simulink library "xpcueilib"  (Simulink 6.0)
settings: Solver=ode45  SolverMode=SingleTasking  StartTime=0.0  StopTime=10.0  RelTol=1e-3
(part 2 of 2)

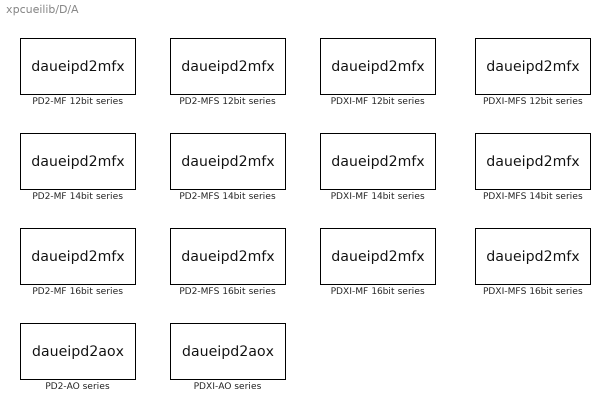
== system xpcueilib/D/A ==
  PD2-AO series : S-Function  InitFcn=muei  FunctionName=daueipd2aox  Parameters=channel, reset, initValue, sampletime, pcislot, boardType, board, devName  mask(ueipd2ao16_da_6){boardtypein=PD2-AO-8/16, channel=[1], reset=[1], initValue=[0], sampletime=0.001, pcislot=-1}
      mask prompts: boardtypein "Board type:"; channel "Channel vector:"; reset "Reset vector:"; initValue "Initial value vector:"; pcislot "PCI slot (-1: autosearch):"
      mask help:
      | PD2-AO series
      | United Electronic Industries
      | Analog Output
      mask init:
      | [board, boardType, devName, reset, initValue, maskdisplay, maskdescription]= mdaueipd2aox(boardtypein, channel, reset, initValue, pcislot);
      | set_param(gcb,'MaskDescription',maskdescription);
      | set_param(gcb,'MaskDisplay',maskdisplay);
      mask Help: helpview(fullfile(docroot, 'mapfiles', 'xpc.map'), 'UEI_PD2-AO-series_DA')
      mask StyleString: popup(PD2-AO-8/16|PD2-AO-16/16|PD2-AO-32/16|PD2-AO-96/16),edit,edit,edit,edit,edit
      mask Display: disp('PD2-AO-8/16\nUEI\nAnalog Output');port_label('input',1,'1');
  PD2-MF 12bit series : S-Function  InitFcn=muei  FunctionName=daueipd2mfx  Parameters=channel, reset, initValue, sampletime, pcislot, boardType, board, devName  mask(ueipd2mf12_da_6){boardtypein=PD2-MF-16-1M/12L, channel=[1], reset=[1], initValue=[0], sampletime=0.001, pcislot=-1}
      mask prompts: boardtypein "Board type:"; channel "Channel vector:"; reset "Reset vector:"; initValue "Initial value vector:"; pcislot "PCI slot (-1: autosearch):"
      mask help:
      | PD2-MF 12bit series
      | United Electronic Industries
      | Analog Output
      mask init: same as xpcueilib/D/A/PD2-AO series
      mask Help: helpview(fullfile(docroot, 'mapfiles', 'xpc.map'), 'UEI_PD2-MF-12bit-series_DA')
      mask StyleString: popup(PD2-MF-16-1M/12L|PD2-MF-16-1M/12H|PD2-MF-64-1M/12L|PD2-MF-64-1M/12H),edit,edit,edit,edit,edit
      mask Display: disp('PD2-MF-16-1M/12L\nUEI\nAnalog Output');port_label('input',1,'1');
  PD2-MF 14bit series : S-Function  InitFcn=muei  FunctionName=daueipd2mfx  Parameters=channel, reset, initValue, sampletime, pcislot, boardType, board, devName  mask(ueipd2mf14_da_6){boardtypein=PD2-MF-16-400/14L, channel=[1], reset=[1], initValue=[0], sampletime=0.001, pcislot=-1}
      mask prompts: boardtypein "Board type:"; channel "Channel vector:"; reset "Reset vector:"; initValue "Initial value vector:"; pcislot "PCI slot (-1: autosearch):"
      mask help:
      | PD2-MF 14bit series
      | United Electronic Industries
      | Analog Output
      mask init: same as xpcueilib/D/A/PD2-AO series
      mask Help: helpview(fullfile(docroot, 'mapfiles', 'xpc.map'), 'UEI_PD2-MF-14bit-series_DA')
      mask StyleString: popup(PD2-MF-16-400/14L|PD2-MF-16-400/14H|PD2-MF-64-400/14L|PD2-MF-64-400/14H|PD2-MF-16-800/14L|PD2-MF-16-800/14H|PD2-MF-64-800/14L|PD2-MF-64-800/14H|PD2-MF-16-2M/14L|PD2-MF-16-2M/14H|PD2-MF-64-2M/14L|PD2-MF-64-2M/14H),edit,edit,edit,edit,edit
      mask Display: disp('PD2-MF-16-400/14L\nUEI\nAnalog Output');port_label('input',1,'1');
  PD2-MF 16bit series : S-Function  InitFcn=muei  FunctionName=daueipd2mfx  Parameters=channel, reset, initValue, sampletime, pcislot, boardType, board, devName  mask(ueipd2mf16_da_6){boardtypein=PD2-MF-16-333/16H, channel=[1], reset=[1], initValue=[0], sampletime=0.001, pcislot=-1}
      mask prompts: boardtypein "Board type:"; channel "Channel vector:"; reset "Reset vector:"; initValue "Initial value vector:"; pcislot "PCI slot (-1: autosearch):"
      mask help:
      | PD2-MF 16bit series
      | United Electronic Industries
      | Analog Output
      mask init: same as xpcueilib/D/A/PD2-AO series
      mask Help: helpview(fullfile(docroot, 'mapfiles', 'xpc.map'), 'UEI_PD2-MF-16bit-series_DA')
      mask StyleString: popup(PD2-MF-16-50/16L|PD2-MF-16-50/16H|PD2-MF-64-50/16L|PD2-MF-64-50/16H|PD2-MF-16-150/16L|PD2-MF-16-150/16H|PD2-MF-64-150/16L|PD2-MF-64-150/16H|PD2-MF-16-333/16L|PD2-MF-16-333/16H|PD2-MF-64-333/16L|PD2-MF-64-333/16H|PD2-MF-16-500/16L|PD2-MF-16-500/16H|PD2-MF-64-500/16L|PD2-MF-64-500/16H),edit,edit,edit,edit,edit
      mask Display: disp('PD2-MF-16-333/16H\nUEI\nAnalog Output');port_label('input',1,'1');
  PD2-MFS 12bit series : S-Function  InitFcn=muei  FunctionName=daueipd2mfx  Parameters=channel, reset, initValue, sampletime, pcislot, boardType, board, devName  mask(ueipd2mfs12_da_6){boardtypein=PD2-MFS-4-1M/12, channel=[1], reset=[1], initValue=[0], sampletime=0.001, pcislot=-1}
      mask prompts: boardtypein "Board type:"; channel "Channel vector:"; reset "Reset vector:"; initValue "Initial value vector:"; pcislot "PCI slot (-1: autosearch):"
      mask help:
      | PD2-MFS 12bit series
      | United Electronic Industries
      | Analog Output
      mask init: same as xpcueilib/D/A/PD2-AO series
      mask Help: helpview(fullfile(docroot, 'mapfiles', 'xpc.map'), 'UEI_PD2-MFS-12bit-series_DA')
      mask StyleString: popup(PD2-MFS-4-1M/12|PD2-MFS-4-1M/12DG|PD2-MFS-4-1M/12H|PD2-MFS-8-1M/12|PD2-MFS-8-1M/12DG|PD2-MFS-8-1M/12H),edit,edit,edit,edit,edit
      mask Display: disp('PD2-MFS-4-1M/12\nUEI\nAnalog Output');port_label('input',1,'1');
  PD2-MFS 14bit series : S-Function  InitFcn=muei  FunctionName=daueipd2mfx  Parameters=channel, reset, initValue, sampletime, pcislot, boardType, board, devName  mask(ueipd2mfs14_da_6){boardtypein=PD2-MFS-4-500/14, channel=[1], reset=[1], initValue=[0], sampletime=0.001, pcislot=-1}
      mask prompts: boardtypein "Board type:"; channel "Channel vector:"; reset "Reset vector:"; initValue "Initial value vector:"; pcislot "PCI slot (-1: autosearch):"
      mask help:
      | PD2-MFS 14bit series
      | United Electronic Industries
      | Analog Output
      mask init: same as xpcueilib/D/A/PD2-AO series
      mask Help: helpview(fullfile(docroot, 'mapfiles', 'xpc.map'), 'UEI_PD2-MFS-14bit-series_DA')
      mask StyleString: popup(PD2-MFS-4-500/14|PD2-MFS-4-500/14DG|PD2-MFS-4-500/14H|PD2-MFS-8-500/14|PD2-MFS-8-500/14DG|PD2-MFS-8-500/14H|PD2-MFS-4-800/14|PD2-MFS-4-800/14DG|PD2-MFS-4-800/14H|PD2-MFS-8-800/14|PD2-MFS-8-800/14DG|PD2-MFS-8-800/14H|PD2-MFS-4-2M/14|PD2-MFS-4-2M/14DG|PD2-MFS-4-2M/14H|PD2-MFS-8-2M/14|PD2-MFS-8-2M/14DG|PD2-MFS-8-2M/14H),edit,edit,edit,edit,edit
      mask Display: disp('PD2-MFS-4-500/14\nUEI\nAnalog Output');port_label('input',1,'1');
  PD2-MFS 16bit series : S-Function  InitFcn=muei  FunctionName=daueipd2mfx  Parameters=channel, reset, initValue, sampletime, pcislot, boardType, board, devName  mask(ueipd2mfs16_da_6){boardtypein=PD2-MFS-4-300/16, channel=[1], reset=[1], initValue=[0], sampletime=0.001, pcislot=-1}
      mask prompts: boardtypein "Board type:"; channel "Channel vector:"; reset "Reset vector:"; initValue "Initial value vector:"; pcislot "PCI slot (-1: autosearch):"
      mask help:
      | PD2-MFS 16bit series
      | United Electronic Industries
      | Analog Output
      mask init: same as xpcueilib/D/A/PD2-AO series
      mask Help: helpview(fullfile(docroot, 'mapfiles', 'xpc.map'), 'UEI_PD2-MFS-16bit-series_DA')
      mask StyleString: popup(PD2-MFS-4-300/16|PD2-MFS-4-300/16DG|PD2-MFS-4-300/16H|PD2-MFS-8-300/16|PD2-MFS-8-300/16DG|PD2-MFS-8-300/16H|PD2-MFS-4-500/16|PD2-MFS-4-500/16DG|PD2-MFS-4-500/16H|PD2-MFS-8-500/16|PD2-MFS-8-500/16DG|PD2-MFS-8-500/16H),edit,edit,edit,edit,edit
      mask Display: disp('PD2-MFS-4-300/16\nUEI\nAnalog Output');port_label('input',1,'1');
  PDXI-AO series : S-Function  InitFcn=muei  FunctionName=daueipd2aox  Parameters=channel, reset, initValue, sampletime, pcislot, boardType, board, devName  mask(ueipdxiao16_da_6){boardtypein=PDXI-AO-8/16, channel=[1], reset=[1], initValue=[0], sampletime=0.001, pcislot=-1}
      mask prompts: boardtypein "Board type:"; channel "Channel vector:"; reset "Reset vector:"; initValue "Initial value vector:"; pcislot "PCI slot (-1: autosearch):"
      mask help:
      | PDXI-AO series
      | United Electronic Industries
      | Analog Output
      mask init: same as xpcueilib/D/A/PD2-AO series
      mask Help: helpview(fullfile(docroot, 'mapfiles', 'xpc.map'), 'UEI_PDXI-AO-series_DA')
      mask StyleString: popup(PDXI-AO-8/16|PDXI-AO-16/16|PDXI-AO-32/16|PDXI-AO-96/16),edit,edit,edit,edit,edit
      mask Display: disp('PDXI-AO-8/16\nUEI\nAnalog Output');port_label('input',1,'1');
  PDXI-MF 12bit series : S-Function  InitFcn=muei  FunctionName=daueipd2mfx  Parameters=channel, reset, initValue, sampletime, pcislot, boardType, board, devName  mask(ueipdximf12_da_6){boardtypein=PDXI-MF-16-1M/12L, channel=[1], reset=[1], initValue=[0], sampletime=0.001, pcislot=-1}
      mask prompts: boardtypein "Board type:"; channel "Channel vector:"; reset "Reset vector:"; initValue "Initial value vector:"; pcislot "PCI slot (-1: autosearch):"
      mask help:
      | PDXI-MF 12bit series
      | United Electronic Industries
      | Analog Output
      mask init: same as xpcueilib/D/A/PD2-AO series
      mask Help: helpview(fullfile(docroot, 'mapfiles', 'xpc.map'), 'UEI_PDXI-MF-12bit-series_DA')
      mask StyleString: popup(PDXI-MF-16-1M/12L|PDXI-MF-16-1M/12H|PDXI-MF-64-1M/12L|PDXI-MF-64-1M/12H),edit,edit,edit,edit,edit
      mask Display: disp('PDXI-MF-16-1M/12L\nUEI\nAnalog Output');port_label('input',1,'1');
  PDXI-MF 14bit series : S-Function  InitFcn=muei  FunctionName=daueipd2mfx  Parameters=channel, reset, initValue, sampletime, pcislot, boardType, board, devName  mask(ueipdximf14_da_6){boardtypein=PDXI-MF-16-400/14L, channel=[1], reset=[1], initValue=[0], sampletime=0.001, pcislot=-1}
      mask prompts: boardtypein "Board type:"; channel "Channel vector:"; reset "Reset vector:"; initValue "Initial value vector:"; pcislot "PCI slot (-1: autosearch):"
      mask help:
      | PDXI-MF 14bit series
      | United Electronic Industries
      | Analog Output
      mask init: same as xpcueilib/D/A/PD2-AO series
      mask Help: helpview(fullfile(docroot, 'mapfiles', 'xpc.map'), 'UEI_PDXI-MF-14bit-series_DA')
      mask StyleString: popup(PDXI-MF-16-400/14L|PDXI-MF-16-400/14H|PDXI-MF-64-400/14L|PDXI-MF-64-400/14H|PDXI-MF-16-800/14L|PDXI-MF-16-800/14H|PDXI-MF-64-800/14L|PDXI-MF-64-800/14H|PDXI-MF-16-2M/14L|PDXI-MF-16-2M/14H|PDXI-MF-64-2M/14L|PDXI-MF-64-2M/14H),edit,edit,edit,edit,edit
      mask Display: disp('PDXI-MF-16-400/14L\nUEI\nAnalog Output');port_label('input',1,'1');
  PDXI-MF 16bit series : S-Function  InitFcn=muei  FunctionName=daueipd2mfx  Parameters=channel, reset, initValue, sampletime, pcislot, boardType, board, devName  mask(ueipdximf16_da_6){boardtypein=PDXI-MF-16-333/16H, channel=[1], reset=[1], initValue=[0], sampletime=0.001, pcislot=-1}
      mask prompts: boardtypein "Board type:"; channel "Channel vector:"; reset "Reset vector:"; initValue "Initial value vector:"; pcislot "PCI slot (-1: autosearch):"
      mask help:
      | PDXI-MF 16bit series
      | United Electronic Industries
      | Analog Output
      mask init: same as xpcueilib/D/A/PD2-AO series
      mask Help: helpview(fullfile(docroot, 'mapfiles', 'xpc.map'), 'UEI_PDXI-MF-16bit-series_DA')
      mask StyleString: popup(PDXI-MF-16-50/16L|PDXI-MF-16-50/16H|PDXI-MF-64-50/16L|PDXI-MF-64-50/16H|PDXI-MF-16-150/16L|PDXI-MF-16-150/16H|PDXI-MF-64-150/16L|PDXI-MF-64-150/16H|PDXI-MF-16-333/16L|PDXI-MF-16-333/16H|PDXI-MF-64-333/16L|PDXI-MF-64-333/16H|PDXI-MF-16-500/16L|PDXI-MF-16-500/16H|PDXI-MF-64-500/16L|PDXI-MF-64-500/16H),edit,edit,edit,edit,edit
      mask Display: disp('PDXI-MF-16-333/16H\nUEI\nAnalog Output');port_label('input',1,'1');
  PDXI-MFS 12bit series : S-Function  InitFcn=muei  FunctionName=daueipd2mfx  Parameters=channel, reset, initValue, sampletime, pcislot, boardType, board, devName  mask(ueipd2mfs12_da_6){boardtypein=PDXI-MFS-4-1M/12, channel=[1], reset=[1], initValue=[0], sampletime=0.001, pcislot=-1}
      mask prompts: boardtypein "Board type:"; channel "Channel vector:"; reset "Reset vector:"; initValue "Initial value vector:"; pcislot "PCI slot (-1: autosearch):"
      mask help:
      | PD2-MFS 12bit series
      | United Electronic Industries
      | Analog Output
      mask init: same as xpcueilib/D/A/PD2-AO series
      mask Help: helpview(fullfile(docroot, 'mapfiles', 'xpc.map'), 'UEI_PDXI-MFS-12bit-series_DA')
      mask StyleString: popup(PDXI-MFS-4-1M/12|PDXI-MFS-4-1M/12DG|PDXI-MFS-4-1M/12H|PDXI-MFS-8-1M/12|PDXI-MFS-8-1M/12DG|PDXI-MFS-8-1M/12H),edit,edit,edit,edit,edit
      mask Display: disp('PDXI-MFS-4-1M/12\nUEI\nAnalog Output');port_label('input',1,'1');
  PDXI-MFS 14bit series : S-Function  InitFcn=muei  FunctionName=daueipd2mfx  Parameters=channel, reset, initValue, sampletime, pcislot, boardType, board, devName  mask(ueipd2mfs14_da_6){boardtypein=PDXI-MFS-4-500/14, channel=[1], reset=[1], initValue=[0], sampletime=0.001, pcislot=-1}
      mask prompts: boardtypein "Board type:"; channel "Channel vector:"; reset "Reset vector:"; initValue "Initial value vector:"; pcislot "PCI slot (-1: autosearch):"
      mask help:
      | PD2-MFS 14bit series
      | United Electronic Industries
      | Analog Output
      mask init: same as xpcueilib/D/A/PD2-AO series
      mask Help: helpview(fullfile(docroot, 'mapfiles', 'xpc.map'), 'UEI_PDXI-MFS-14bit-series_DA')
      mask StyleString: popup(PDXI-MFS-4-500/14|PDXI-MFS-4-500/14DG|PDXI-MFS-4-500/14H|PDXI-MFS-8-500/14|PDXI-MFS-8-500/14DG|PDXI-MFS-8-500/14H|PDXI-MFS-4-800/14|PDXI-MFS-4-800/14DG|PDXI-MFS-4-800/14H|PDXI-MFS-8-800/14|PDXI-MFS-8-800/14DG|PDXI-MFS-8-800/14H|PDXI-MFS-4-2M/14|PDXI-MFS-4-2M/14DG|PDXI-MFS-4-2M/14H|PDXI-MFS-8-2M/14|PDXI-MFS-8-2M/14DG|PDXI-MFS-8-2M/14H),edit,edit,edit,edit,edit
      mask Display: disp('PDXI-MFS-4-500/14\nUEI\nAnalog Output');port_label('input',1,'1');
  PDXI-MFS 16bit series : S-Function  InitFcn=muei  FunctionName=daueipd2mfx  Parameters=channel, reset, initValue, sampletime, pcislot, boardType, board, devName  mask(ueipd2mfs16_da_6){boardtypein=PDXI-MFS-4-300/16, channel=[1], reset=[1], initValue=[0], sampletime=0.001, pcislot=-1}
      mask prompts: boardtypein "Board type:"; channel "Channel vector:"; reset "Reset vector:"; initValue "Initial value vector:"; pcislot "PCI slot (-1: autosearch):"
      mask help:
      | PD2-MFS 16bit series
      | United Electronic Industries
      | Analog Output
      mask init: same as xpcueilib/D/A/PD2-AO series
      mask Help: helpview(fullfile(docroot, 'mapfiles', 'xpc.map'), 'UEI_PDXI-MFS-16bit-series_DA')
      mask StyleString: popup(PDXI-MFS-4-300/16|PDXI-MFS-4-300/16DG|PDXI-MFS-4-300/16H|PDXI-MFS-8-300/16|PDXI-MFS-8-300/16DG|PDXI-MFS-8-300/16H|PDXI-MFS-4-500/16|PDXI-MFS-4-500/16DG|PDXI-MFS-4-500/16H|PDXI-MFS-8-500/16|PDXI-MFS-8-500/16DG|PDXI-MFS-8-500/16H),edit,edit,edit,edit,edit
      mask Display: disp('PDXI-MFS-4-300/16\nUEI\nAnalog Output');port_label('input',1,'1');

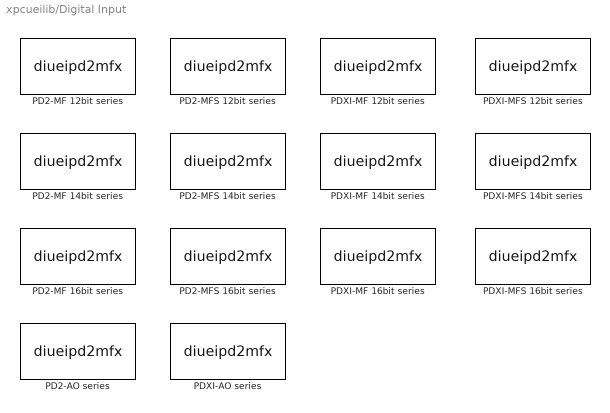
== system xpcueilib/Digital Input ==
  PD2-AO series : S-Function  InitFcn=muei  FunctionName=diueipd2mfx  Parameters=channel, sampletime, pcislot, boardType, board, devName  mask(ueipd2ao16_di_4){boardtypein=PD2-AO-8/16, channel=[1], sampletime=0.001, pcislot=-1}
      mask prompts: boardtypein "Board type:"; channel "Channel vector:"; pcislot "PCI slot (-1: autosearch):"
      mask help:
      | PD2-AO series
      | United Electronic Industries
      | Digital Input
      mask init:
      | [board, boardType, devName, maskdisplay, maskdescription]= mdiuei(boardtypein, channel, pcislot);
      | set_param(gcb,'MaskDescription',maskdescription);
      | set_param(gcb,'MaskDisplay',maskdisplay);
      mask Help: helpview(fullfile(docroot, 'mapfiles', 'xpc.map'), 'UEI_PD2-AO-series_DIN')
      mask StyleString: popup(PD2-AO-8/16|PD2-AO-16/16|PD2-AO-32/16),edit,edit,edit
      mask Display: disp('PD2-AO-8/16\nUEI\nDigital Input');port_label('output',1,'1');
  PD2-MF 12bit series : S-Function  InitFcn=muei  FunctionName=diueipd2mfx  Parameters=channel, sampletime, pcislot, boardType, board, devName  mask(ueipd2mf12_di_4){boardtypein=PD2-MF-16-1M/12L, channel=[1], sampletime=0.001, pcislot=-1}
      mask prompts: boardtypein "Board type:"; channel "Channel vector:"; pcislot "PCI slot (-1: autosearch):"
      mask help:
      | PD2-MF 12bit series
      | United Electronic Industries
      | Digital Input
      mask init:
      | [board, boardType, devName, maskdisplay, maskdescription]= mdiuei(boardtypein, channel, pcislot);
      | set_param(gcb,'MaskDescription',maskdescription);
      | set_param(gcb,'MaskDisplay',maskdisplay);
      mask Help: helpview(fullfile(docroot, 'mapfiles', 'xpc.map'), 'UEI_PD2-MF-12bit-series_DIN')
      mask StyleString: popup(PD2-MF-16-1M/12L|PD2-MF-16-1M/12H|PD2-MF-64-1M/12L|PD2-MF-64-1M/12H),edit,edit,edit
      mask Display: disp('PD2-MF-16-1M/12L\nUEI\nDigital Input');port_label('output',1,'1');
  PD2-MF 14bit series : S-Function  InitFcn=muei  FunctionName=diueipd2mfx  Parameters=channel, sampletime, pcislot, boardType, board, devName  mask(ueipd2mf14_di_4){boardtypein=PD2-MF-16-400/14L, channel=[1], sampletime=0.001, pcislot=-1}
      mask prompts: boardtypein "Board type:"; channel "Channel vector:"; pcislot "PCI slot (-1: autosearch):"
      mask help:
      | PD2-MF 14bit series
      | United Electronic Industries
      | Digital Input
      mask init:
      | [board, boardType, devName, maskdisplay, maskdescription]= mdiuei(boardtypein, channel, pcislot);
      | set_param(gcb,'MaskDescription',maskdescription);
      | set_param(gcb,'MaskDisplay',maskdisplay);
      mask Help: helpview(fullfile(docroot, 'mapfiles', 'xpc.map'), 'UEI_PD2-MF-14bit-series_DIN')
      mask StyleString: popup(PD2-MF-16-400/14L|PD2-MF-16-400/14H|PD2-MF-64-400/14L|PD2-MF-64-400/14H|PD2-MF-16-800/14L|PD2-MF-16-800/14H|PD2-MF-64-800/14L|PD2-MF-64-800/14H|PD2-MF-16-2M/14L|PD2-MF-16-2M/14H|PD2-MF-64-2M/14L|PD2-MF-64-2M/14H),edit,edit,edit
      mask Display: disp('PD2-MF-16-400/14L\nUEI\nDigital Input');port_label('output',1,'1');
  PD2-MF 16bit series : S-Function  InitFcn=muei  FunctionName=diueipd2mfx  Parameters=channel, sampletime, pcislot, boardType, board, devName  mask(ueipd2mf16_di_4){boardtypein=PD2-MF-16-333/16H, channel=[1], sampletime=0.001, pcislot=-1}
      mask prompts: boardtypein "Board type:"; channel "Channel vector:"; pcislot "PCI slot (-1: autosearch):"
      mask help:
      | PD2-MF 16bit series
      | United Electronic Industries
      | Digital Input
      mask init:
      | [board, boardType, devName, maskdisplay, maskdescription]= mdiuei(boardtypein, channel, pcislot);
      | set_param(gcb,'MaskDescription',maskdescription);
      | set_param(gcb,'MaskDisplay',maskdisplay);
      mask Help: helpview(fullfile(docroot, 'mapfiles', 'xpc.map'), 'UEI_PD2-MF-16bit-series_DIN')
      mask StyleString: popup(PD2-MF-16-50/16L|PD2-MF-16-50/16H|PD2-MF-64-50/16L|PD2-MF-64-50/16H|PD2-MF-16-150/16L|PD2-MF-16-150/16H|PD2-MF-64-150/16L|PD2-MF-64-150/16H|PD2-MF-16-333/16L|PD2-MF-16-333/16H|PD2-MF-64-333/16L|PD2-MF-64-333/16H|PD2-MF-16-500/16L|PD2-MF-16-500/16H|PD2-MF-64-500/16L|PD2-MF-64-500/16H),edit,edit,edit
      mask Display: disp('PD2-MF-16-333/16H\nUEI\nDigital Input');port_label('output',1,'1');
  PD2-MFS 12bit series : S-Function  InitFcn=muei  FunctionName=diueipd2mfx  Parameters=channel, sampletime, pcislot, boardType, board, devName  mask(ueipd2mfs12_di_4){boardtypein=PD2-MFS-4-1M/12, channel=[1], sampletime=0.001, pcislot=-1}
      mask prompts: boardtypein "Board type:"; channel "Channel vector:"; pcislot "PCI slot (-1: autosearch):"
      mask help:
      | PD2-MFS 12bit series
      | United Electronic Industries
      | Digital Input
      mask init:
      | [board, boardType, devName, maskdisplay, maskdescription]= mdiuei(boardtypein, channel, pcislot);
      | set_param(gcb,'MaskDescription',maskdescription);
      | set_param(gcb,'MaskDisplay',maskdisplay);
      mask Help: helpview(fullfile(docroot, 'mapfiles', 'xpc.map'), 'UEI_PD2-MFS-12bit-series_DIN')
      mask StyleString: popup(PD2-MFS-4-1M/12|PD2-MFS-4-1M/12DG|PD2-MFS-4-1M/12H|PD2-MFS-8-1M/12|PD2-MFS-8-1M/12DG|PD2-MFS-8-1M/12H),edit,edit,edit
      mask Display: disp('PD2-MFS-4-1M/12\nUEI\nDigital Input');port_label('output',1,'1');
  PD2-MFS 14bit series : S-Function  InitFcn=muei  FunctionName=diueipd2mfx  Parameters=channel, sampletime, pcislot, boardType, board, devName  mask(ueipd2mfs14_di_4){boardtypein=PD2-MFS-4-500/14, channel=[1], sampletime=0.001, pcislot=-1}
      mask prompts: boardtypein "Board type:"; channel "Channel vector:"; pcislot "PCI slot (-1: autosearch):"
      mask help:
      | PD2-MFS 14bit series
      | United Electronic Industries
      | Digital Input
      mask init:
      | [board, boardType, devName, maskdisplay, maskdescription]= mdiuei(boardtypein, channel, pcislot);
      | set_param(gcb,'MaskDescription',maskdescription);
      | set_param(gcb,'MaskDisplay',maskdisplay);
      mask Help: helpview(fullfile(docroot, 'mapfiles', 'xpc.map'), 'UEI_PD2-MFS-14bit-series_DIN')
      mask StyleString: popup(PD2-MFS-4-500/14|PD2-MFS-4-500/14DG|PD2-MFS-4-500/14H|PD2-MFS-8-500/14|PD2-MFS-8-500/14DG|PD2-MFS-8-500/14H|PD2-MFS-4-800/14|PD2-MFS-4-800/14DG|PD2-MFS-4-800/14H|PD2-MFS-8-800/14|PD2-MFS-8-800/14DG|PD2-MFS-8-800/14H|PD2-MFS-4-2M/14|PD2-MFS-4-2M/14DG|PD2-MFS-4-2M/14H|PD2-MFS-8-2M/14|PD2-MFS-8-2M/14DG|PD2-MFS-8-2M/14H),edit,edit,edit
      mask Display: disp('PD2-MFS-4-500/14\nUEI\nDigital Input');port_label('output',1,'1');
  PD2-MFS 16bit series : S-Function  InitFcn=muei  FunctionName=diueipd2mfx  Parameters=channel, sampletime, pcislot, boardType, board, devName  mask(ueipd2mfs16_di_4){boardtypein=PD2-MFS-4-300/16, channel=[1], sampletime=0.001, pcislot=-1}
      mask prompts: boardtypein "Board type:"; channel "Channel vector:"; pcislot "PCI slot (-1: autosearch):"
      mask help:
      | PD2-MFS 16bit series
      | United Electronic Industries
      | Digital Input
      mask init:
      | [board, boardType, devName, maskdisplay, maskdescription]= mdiuei(boardtypein, channel, pcislot);
      | set_param(gcb,'MaskDescription',maskdescription);
      | set_param(gcb,'MaskDisplay',maskdisplay);
      mask Help: helpview(fullfile(docroot, 'mapfiles', 'xpc.map'), 'UEI_PD2-MFS-16bit-series_DIN')
      mask StyleString: popup(PD2-MFS-4-300/16|PD2-MFS-4-300/16DG|PD2-MFS-4-300/16H|PD2-MFS-8-300/16|PD2-MFS-8-300/16DG|PD2-MFS-8-300/16H|PD2-MFS-4-500/16|PD2-MFS-4-500/16DG|PD2-MFS-4-500/16H|PD2-MFS-8-500/16|PD2-MFS-8-500/16DG|PD2-MFS-8-500/16H),edit,edit,edit
      mask Display: disp('PD2-MFS-4-300/16\nUEI\nDigital Input');port_label('output',1,'1');
  PDXI-AO series : S-Function  InitFcn=muei  FunctionName=diueipd2mfx  Parameters=channel, sampletime, pcislot, boardType, board, devName  mask(ueipdxiao16_di_4){boardtypein=PDXI-AO-8/16, channel=[1], sampletime=0.001, pcislot=-1}
      mask prompts: boardtypein "Board type:"; channel "Channel vector:"; pcislot "PCI slot (-1: autosearch):"
      mask help:
      | PDXI-AO series
      | United Electronic Industries
      | Digital Input
      mask init:
      | [board, boardType, devName, maskdisplay, maskdescription]= mdiuei(boardtypein, channel, pcislot);
      | set_param(gcb,'MaskDescription',maskdescription);
      | set_param(gcb,'MaskDisplay',maskdisplay);
      mask Help: helpview(fullfile(docroot, 'mapfiles', 'xpc.map'), 'UEI_PDXI-AO-series_DIN')
      mask StyleString: popup(PDXI-AO-8/16|PDXI-AO-16/16|PDXI-AO-32/16),edit,edit,edit
      mask Display: disp('PDXI-AO-8/16\nUEI\nDigital Input');port_label('output',1,'1');
  PDXI-MF 12bit series : S-Function  InitFcn=muei  FunctionName=diueipd2mfx  Parameters=channel, sampletime, pcislot, boardType, board, devName  mask(ueipdximf12_di_4){boardtypein=PDXI-MF-16-1M/12L, channel=[1], sampletime=0.001, pcislot=-1}
      mask prompts: boardtypein "Board type:"; channel "Channel vector:"; pcislot "PCI slot (-1: autosearch):"
      mask help:
      | PDXI-MF 12bit series
      | United Electronic Industries
      | Digital Input
      mask init:
      | [board, boardType, devName, maskdisplay, maskdescription]= mdiuei(boardtypein, channel, pcislot);
      | set_param(gcb,'MaskDescription',maskdescription);
      | set_param(gcb,'MaskDisplay',maskdisplay);
      mask Help: helpview(fullfile(docroot, 'mapfiles', 'xpc.map'), 'UEI_PDXI-MF-12bit-series_DIN')
      mask StyleString: popup(PDXI-MF-16-1M/12L|PDXI-MF-16-1M/12H|PDXI-MF-64-1M/12L|PDXI-MF-64-1M/12H),edit,edit,edit
      mask Display: disp('PDXI-MF-16-1M/12L\nUEI\nDigital Input');port_label('output',1,'1');
  PDXI-MF 14bit series : S-Function  InitFcn=muei  FunctionName=diueipd2mfx  Parameters=channel, sampletime, pcislot, boardType, board, devName  mask(ueipdximf14_di_4){boardtypein=PDXI-MF-16-400/14L, channel=[1], sampletime=0.001, pcislot=-1}
      mask prompts: boardtypein "Board type:"; channel "Channel vector:"; pcislot "PCI slot (-1: autosearch):"
      mask help:
      | PDXI-MF 14bit series
      | United Electronic Industries
      | Digital Input
      mask init:
      | [board, boardType, devName, maskdisplay, maskdescription]= mdiuei(boardtypein, channel, pcislot);
      | set_param(gcb,'MaskDescription',maskdescription);
      | set_param(gcb,'MaskDisplay',maskdisplay);
      mask Help: helpview(fullfile(docroot, 'mapfiles', 'xpc.map'), 'UEI_PDXI-MF-14bit-series_DIN')
      mask StyleString: popup(PDXI-MF-16-400/14L|PDXI-MF-16-400/14H|PDXI-MF-64-400/14L|PDXI-MF-64-400/14H|PDXI-MF-16-800/14L|PDXI-MF-16-800/14H|PDXI-MF-64-800/14L|PDXI-MF-64-800/14H|PDXI-MF-16-2M/14L|PDXI-MF-16-2M/14H|PDXI-MF-64-2M/14L|PDXI-MF-64-2M/14H),edit,edit,edit
      mask Display: disp('PDXI-MF-16-400/14L\nUEI\nDigital Input');port_label('output',1,'1');
  PDXI-MF 16bit series : S-Function  InitFcn=muei  FunctionName=diueipd2mfx  Parameters=channel, sampletime, pcislot, boardType, board, devName  mask(ueipdximf16_di_4){boardtypein=PDXI-MF-16-333/16H, channel=[1], sampletime=0.001, pcislot=-1}
      mask prompts: boardtypein "Board type:"; channel "Channel vector:"; pcislot "PCI slot (-1: autosearch):"
      mask help:
      | PDXI-MF 16bit series
      | United Electronic Industries
      | Digital Input
      mask init:
      | [board, boardType, devName, maskdisplay, maskdescription]= mdiuei(boardtypein, channel, pcislot);
      | set_param(gcb,'MaskDescription',maskdescription);
      | set_param(gcb,'MaskDisplay',maskdisplay);
      mask Help: helpview(fullfile(docroot, 'mapfiles', 'xpc.map'), 'UEI_PDXI-MF-16bit-series_DIN')
      mask StyleString: popup(PDXI-MF-16-50/16L|PDXI-MF-16-50/16H|PDXI-MF-64-50/16L|PDXI-MF-64-50/16H|PDXI-MF-16-150/16L|PDXI-MF-16-150/16H|PDXI-MF-64-150/16L|PDXI-MF-64-150/16H|PDXI-MF-16-333/16L|PDXI-MF-16-333/16H|PDXI-MF-64-333/16L|PDXI-MF-64-333/16H|PDXI-MF-16-500/16L|PDXI-MF-16-500/16H|PDXI-MF-64-500/16L|PDXI-MF-64-500/16H),edit,edit,edit
      mask Display: disp('PDXI-MF-16-333/16H\nUEI\nDigital Input');port_label('output',1,'1');
  PDXI-MFS 12bit series : S-Function  InitFcn=muei  FunctionName=diueipd2mfx  Parameters=channel, sampletime, pcislot, boardType, board, devName  mask(ueipd2mfs12_di_4){boardtypein=PDXI-MFS-4-1M/12, channel=[1], sampletime=0.001, pcislot=-1}
      mask prompts: boardtypein "Board type:"; channel "Channel vector:"; pcislot "PCI slot (-1: autosearch):"
      mask help:
      | PD2-MFS 12bit series
      | United Electronic Industries
      | Digital Input
      mask init:
      | [board, boardType, devName, maskdisplay, maskdescription]= mdiuei(boardtypein, channel, pcislot);
      | set_param(gcb,'MaskDescription',maskdescription);
      | set_param(gcb,'MaskDisplay',maskdisplay);
      mask Help: helpview(fullfile(docroot, 'mapfiles', 'xpc.map'), 'UEI_PDXI-MFS-12bit-series_DIN')
      mask StyleString: popup(PDXI-MFS-4-1M/12|PDXI-MFS-4-1M/12DG|PDXI-MFS-4-1M/12H|PDXI-MFS-8-1M/12|PDXI-MFS-8-1M/12DG|PDXI-MFS-8-1M/12H),edit,edit,edit
      mask Display: disp('PDXI-MFS-4-1M/12\nUEI\nDigital Input');port_label('output',1,'1');
  PDXI-MFS 14bit series : S-Function  InitFcn=muei  FunctionName=diueipd2mfx  Parameters=channel, sampletime, pcislot, boardType, board, devName  mask(ueipd2mfs14_di_4){boardtypein=PDXI-MFS-4-500/14, channel=[1], sampletime=0.001, pcislot=-1}
      mask prompts: boardtypein "Board type:"; channel "Channel vector:"; pcislot "PCI slot (-1: autosearch):"
      mask help:
      | PD2-MFS 14bit series
      | United Electronic Industries
      | Digital Input
      mask init:
      | [board, boardType, devName, maskdisplay, maskdescription]= mdiuei(boardtypein, channel, pcislot);
      | set_param(gcb,'MaskDescription',maskdescription);
      | set_param(gcb,'MaskDisplay',maskdisplay);
      mask Help: helpview(fullfile(docroot, 'mapfiles', 'xpc.map'), 'UEI_PDXI-MFS-14bit-series_DIN')
      mask StyleString: popup(PDXI-MFS-4-500/14|PDXI-MFS-4-500/14DG|PDXI-MFS-4-500/14H|PDXI-MFS-8-500/14|PDXI-MFS-8-500/14DG|PDXI-MFS-8-500/14H|PDXI-MFS-4-800/14|PDXI-MFS-4-800/14DG|PDXI-MFS-4-800/14H|PDXI-MFS-8-800/14|PDXI-MFS-8-800/14DG|PDXI-MFS-8-800/14H|PDXI-MFS-4-2M/14|PDXI-MFS-4-2M/14DG|PDXI-MFS-4-2M/14H|PDXI-MFS-8-2M/14|PDXI-MFS-8-2M/14DG|PDXI-MFS-8-2M/14H),edit,edit,edit
      mask Display: disp('PDXI-MFS-4-500/14\nUEI\nDigital Input');port_label('output',1,'1');
  PDXI-MFS 16bit series : S-Function  InitFcn=muei  FunctionName=diueipd2mfx  Parameters=channel, sampletime, pcislot, boardType, board, devName  mask(ueipd2mfs16_di_4){boardtypein=PDXI-MFS-4-300/16, channel=[1], sampletime=0.001, pcislot=-1}
      mask prompts: boardtypein "Board type:"; channel "Channel vector:"; pcislot "PCI slot (-1: autosearch):"
      mask help:
      | PD2-MFS 16bit series
      | United Electronic Industries
      | Digital Input
      mask init:
      | [board, boardType, devName, maskdisplay, maskdescription]= mdiuei(boardtypein, channel, pcislot);
      | set_param(gcb,'MaskDescription',maskdescription);
      | set_param(gcb,'MaskDisplay',maskdisplay);
      mask Help: helpview(fullfile(docroot, 'mapfiles', 'xpc.map'), 'UEI_PDXI-MFS-16bit-series_DIN')
      mask StyleString: popup(PDXI-MFS-4-300/16|PDXI-MFS-4-300/16DG|PDXI-MFS-4-300/16H|PDXI-MFS-8-300/16|PDXI-MFS-8-300/16DG|PDXI-MFS-8-300/16H|PDXI-MFS-4-500/16|PDXI-MFS-4-500/16DG|PDXI-MFS-4-500/16H|PDXI-MFS-8-500/16|PDXI-MFS-8-500/16DG|PDXI-MFS-8-500/16H),edit,edit,edit
      mask Display: disp('PDXI-MFS-4-300/16\nUEI\nDigital Input');port_label('output',1,'1');

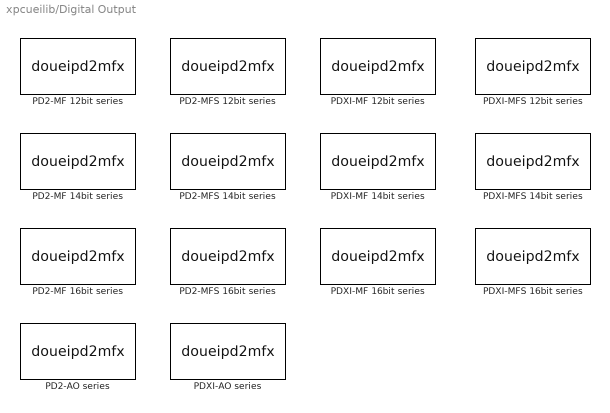
== system xpcueilib/Digital Output ==
  PD2-AO series : S-Function  InitFcn=muei  FunctionName=doueipd2mfx  Parameters=channel, reset, initValue, sampletime, pcislot, boardType, board, devName  mask(ueipd2ao16_do_6){boardtypein=PD2-AO-8/16, channel=[1], reset=[1], initValue=[0], sampletime=0.001, pcislot=-1}
      mask prompts: boardtypein "Board type:"; channel "Channel vector:"; reset "Reset vector:"; initValue "Initial value vector:"; pcislot "PCI slot (-1: autosearch):"
      mask help:
      | PD2-AO series
      | United Electronic Industries
      | Digital Output
      mask init:
      | [board, boardType, devName, reset, initValue, maskdisplay, maskdescription]= mdouei(boardtypein, channel, reset, initValue, pcislot);
      | set_param(gcb,'MaskDescription',maskdescription);
      | set_param(gcb,'MaskDisplay',maskdisplay);
      mask Help: helpview(fullfile(docroot, 'mapfiles', 'xpc.map'), 'UEI_PD2-AO-series_DOUT')
      mask StyleString: popup(PD2-AO-8/16|PD2-AO-16/16|PD2-AO-32/16),edit,edit,edit,edit,edit
      mask Display: disp('PD2-AO-8/16\nUEI\nDigital Output');port_label('input',1,'1');
  PD2-MF 12bit series : S-Function  InitFcn=muei  FunctionName=doueipd2mfx  Parameters=channel, reset, initValue, sampletime, pcislot, boardType, board, devName  mask(ueipd2mf12_do_6){boardtypein=PD2-MF-16-1M/12L, channel=[1], reset=[1], initValue=[0], sampletime=0.001, pcislot=-1}
      mask prompts: boardtypein "Board type:"; channel "Channel vector:"; reset "Reset vector:"; initValue "Initial value vector:"; pcislot "PCI slot (-1: autosearch):"
      mask help:
      | PD2-MF 12bit series
      | United Electronic Industries
      | Digital Output
      mask init: same as xpcueilib/Digital Output/PD2-AO series
      mask Help: helpview(fullfile(docroot, 'mapfiles', 'xpc.map'), 'UEI_PD2-MF-12bit-series_DOUT')
      mask StyleString: popup(PD2-MF-16-1M/12L|PD2-MF-16-1M/12H|PD2-MF-64-1M/12L|PD2-MF-64-1M/12H),edit,edit,edit,edit,edit
      mask Display: disp('PD2-MF-16-1M/12L\nUEI\nDigital Output');port_label('input',1,'1');
  PD2-MF 14bit series : S-Function  InitFcn=muei  FunctionName=doueipd2mfx  Parameters=channel, reset, initValue, sampletime, pcislot, boardType, board, devName  mask(ueipd2mf14_do_6){boardtypein=PD2-MF-16-400/14L, channel=[1], reset=[1], initValue=[0], sampletime=0.001, pcislot=-1}
      mask prompts: boardtypein "Board type:"; channel "Channel vector:"; reset "Reset vector:"; initValue "Initial value vector:"; pcislot "PCI slot (-1: autosearch):"
      mask help:
      | PD2-MF 14bit series
      | United Electronic Industries
      | Digital Output
      mask init: same as xpcueilib/Digital Output/PD2-AO series
      mask Help: helpview(fullfile(docroot, 'mapfiles', 'xpc.map'), 'UEI_PD2-MF-14bit-series_DOUT')
      mask StyleString: popup(PD2-MF-16-400/14L|PD2-MF-16-400/14H|PD2-MF-64-400/14L|PD2-MF-64-400/14H|PD2-MF-16-800/14L|PD2-MF-16-800/14H|PD2-MF-64-800/14L|PD2-MF-64-800/14H|PD2-MF-16-2M/14L|PD2-MF-16-2M/14H|PD2-MF-64-2M/14L|PD2-MF-64-2M/14H),edit,edit,edit,edit,edit
      mask Display: disp('PD2-MF-16-400/14L\nUEI\nDigital Output');port_label('input',1,'1');
  PD2-MF 16bit series : S-Function  InitFcn=muei  FunctionName=doueipd2mfx  Parameters=channel, reset, initValue, sampletime, pcislot, boardType, board, devName  mask(ueipd2mf16_do_6){boardtypein=PD2-MF-16-333/16H, channel=[1], reset=[1], initValue=[0], sampletime=0.001, pcislot=-1}
      mask prompts: boardtypein "Board type:"; channel "Channel vector:"; reset "Reset vector:"; initValue "Initial value vector:"; pcislot "PCI slot (-1: autosearch):"
      mask help:
      | PD2-MF 16bit series
      | United Electronic Industries
      | Digital Output
      mask init: same as xpcueilib/Digital Output/PD2-AO series
      mask Help: helpview(fullfile(docroot, 'mapfiles', 'xpc.map'), 'UEI_PD2-MF-16bit-series_DOUT')
      mask StyleString: popup(PD2-MF-16-50/16L|PD2-MF-16-50/16H|PD2-MF-64-50/16L|PD2-MF-64-50/16H|PD2-MF-16-150/16L|PD2-MF-16-150/16H|PD2-MF-64-150/16L|PD2-MF-64-150/16H|PD2-MF-16-333/16L|PD2-MF-16-333/16H|PD2-MF-64-333/16L|PD2-MF-64-333/16H|PD2-MF-16-500/16L|PD2-MF-16-500/16H|PD2-MF-64-500/16L|PD2-MF-64-500/16H),edit,edit,edit,edit,edit
      mask Display: disp('PD2-MF-16-333/16H\nUEI\nDigital Output');port_label('input',1,'1');
  PD2-MFS 12bit series : S-Function  InitFcn=muei  FunctionName=doueipd2mfx  Parameters=channel, reset, initValue, sampletime, pcislot, boardType, board, devName  mask(ueipd2mfs12_do_6){boardtypein=PD2-MFS-4-1M/12, channel=[1], reset=[1], initValue=[0], sampletime=0.001, pcislot=-1}
      mask prompts: boardtypein "Board type:"; channel "Channel vector:"; reset "Reset vector:"; initValue "Initial value vector:"; pcislot "PCI slot (-1: autosearch):"
      mask help:
      | PD2-MFS 12bit series
      | United Electronic Industries
      | Digital Output
      mask init: same as xpcueilib/Digital Output/PD2-AO series
      mask Help: helpview(fullfile(docroot, 'mapfiles', 'xpc.map'), 'UEI_PD2-MFS-12bit-series_DOUT')
      mask StyleString: popup(PD2-MFS-4-1M/12|PD2-MFS-4-1M/12DG|PD2-MFS-4-1M/12H|PD2-MFS-8-1M/12|PD2-MFS-8-1M/12DG|PD2-MFS-8-1M/12H),edit,edit,edit,edit,edit
      mask Display: disp('PD2-MFS-4-1M/12\nUEI\nDigital Output');port_label('input',1,'1');
  PD2-MFS 14bit series : S-Function  InitFcn=muei  FunctionName=doueipd2mfx  Parameters=channel, reset, initValue, sampletime, pcislot, boardType, board, devName  mask(ueipd2mfs14_do_6){boardtypein=PD2-MFS-4-500/14, channel=[1], reset=[1], initValue=[0], sampletime=0.001, pcislot=-1}
      mask prompts: boardtypein "Board type:"; channel "Channel vector:"; reset "Reset vector:"; initValue "Initial value vector:"; pcislot "PCI slot (-1: autosearch):"
      mask help:
      | PD2-MFS 14bit series
      | United Electronic Industries
      | Digital Output
      mask init: same as xpcueilib/Digital Output/PD2-AO series
      mask Help: helpview(fullfile(docroot, 'mapfiles', 'xpc.map'), 'UEI_PD2-MFS-14bit-series_DOUT')
      mask StyleString: popup(PD2-MFS-4-500/14|PD2-MFS-4-500/14DG|PD2-MFS-4-500/14H|PD2-MFS-8-500/14|PD2-MFS-8-500/14DG|PD2-MFS-8-500/14H|PD2-MFS-4-800/14|PD2-MFS-4-800/14DG|PD2-MFS-4-800/14H|PD2-MFS-8-800/14|PD2-MFS-8-800/14DG|PD2-MFS-8-800/14H|PD2-MFS-4-2M/14|PD2-MFS-4-2M/14DG|PD2-MFS-4-2M/14H|PD2-MFS-8-2M/14|PD2-MFS-8-2M/14DG|PD2-MFS-8-2M/14H),edit,edit,edit,edit,edit
      mask Display: disp('PD2-MFS-4-500/14\nUEI\nDigital Output');port_label('input',1,'1');
  PD2-MFS 16bit series : S-Function  InitFcn=muei  FunctionName=doueipd2mfx  Parameters=channel, reset, initValue, sampletime, pcislot, boardType, board, devName  mask(ueipd2mfs16_do_6){boardtypein=PD2-MFS-4-300/16, channel=[1], reset=[1], initValue=[0], sampletime=0.001, pcislot=-1}
      mask prompts: boardtypein "Board type:"; channel "Channel vector:"; reset "Reset vector:"; initValue "Initial value vector:"; pcislot "PCI slot (-1: autosearch):"
      mask help:
      | PD2-MFS 16bit series
      | United Electronic Industries
      | Digital Output
      mask init: same as xpcueilib/Digital Output/PD2-AO series
      mask Help: helpview(fullfile(docroot, 'mapfiles', 'xpc.map'), 'UEI_PD2-MFS-16bit-series_DOUT')
      mask StyleString: popup(PD2-MFS-4-300/16|PD2-MFS-4-300/16DG|PD2-MFS-4-300/16H|PD2-MFS-8-300/16|PD2-MFS-8-300/16DG|PD2-MFS-8-300/16H|PD2-MFS-4-500/16|PD2-MFS-4-500/16DG|PD2-MFS-4-500/16H|PD2-MFS-8-500/16|PD2-MFS-8-500/16DG|PD2-MFS-8-500/16H),edit,edit,edit,edit,edit
      mask Display: disp('PD2-MFS-4-300/16\nUEI\nDigital Output');port_label('input',1,'1');
  PDXI-AO series : S-Function  InitFcn=muei  FunctionName=doueipd2mfx  Parameters=channel, reset, initValue, sampletime, pcislot, boardType, board, devName  mask(ueipdxiao16_do_6){boardtypein=PDXI-AO-8/16, channel=[1], reset=[1], initValue=[0], sampletime=0.001, pcislot=-1}
      mask prompts: boardtypein "Board type:"; channel "Channel vector:"; reset "Reset vector:"; initValue "Initial value vector:"; pcislot "PCI slot (-1: autosearch):"
      mask help:
      | PDXI-AO series
      | United Electronic Industries
      | Digital Output
      mask init: same as xpcueilib/Digital Output/PD2-AO series
      mask Help: helpview(fullfile(docroot, 'mapfiles', 'xpc.map'), 'UEI_PDXI-AO-series_DOUT')
      mask StyleString: popup(PDXI-AO-8/16|PDXI-AO-16/16|PDXI-AO-32/16),edit,edit,edit,edit,edit
      mask Display: disp('PDXI-AO-8/16\nUEI\nDigital Output');port_label('input',1,'1');
  PDXI-MF 12bit series : S-Function  InitFcn=muei  FunctionName=doueipd2mfx  Parameters=channel, reset, initValue, sampletime, pcislot, boardType, board, devName  mask(ueipdximf12_do_6){boardtypein=PDXI-MF-16-1M/12L, channel=[1], reset=[1], initValue=[0], sampletime=0.001, pcislot=-1}
      mask prompts: boardtypein "Board type:"; channel "Channel vector:"; reset "Reset vector:"; initValue "Initial value vector:"; pcislot "PCI slot (-1: autosearch):"
      mask help:
      | PDXI-MF 12bit series
      | United Electronic Industries
      | Digital Output
      mask init: same as xpcueilib/Digital Output/PD2-AO series
      mask Help: helpview(fullfile(docroot, 'mapfiles', 'xpc.map'), 'UEI_PDXI-MF-12bit-series_DOUT')
      mask StyleString: popup(PDXI-MF-16-1M/12L|PDXI-MF-16-1M/12H|PDXI-MF-64-1M/12L|PDXI-MF-64-1M/12H),edit,edit,edit,edit,edit
      mask Display: disp('PDXI-MF-16-1M/12L\nUEI\nDigital Output');port_label('input',1,'1');
  PDXI-MF 14bit series : S-Function  InitFcn=muei  FunctionName=doueipd2mfx  Parameters=channel, reset, initValue, sampletime, pcislot, boardType, board, devName  mask(ueipdximf14_do_6){boardtypein=PDXI-MF-16-400/14L, channel=[1], reset=[1], initValue=[0], sampletime=0.001, pcislot=-1}
      mask prompts: boardtypein "Board type:"; channel "Channel vector:"; reset "Reset vector:"; initValue "Initial value vector:"; pcislot "PCI slot (-1: autosearch):"
      mask help:
      | PDXI-MF 14bit series
      | United Electronic Industries
      | Digital Output
      mask init: same as xpcueilib/Digital Output/PD2-AO series
      mask Help: helpview(fullfile(docroot, 'mapfiles', 'xpc.map'), 'UEI_PDXI-MF-14bit-series_DOUT')
      mask StyleString: popup(PDXI-MF-16-400/14L|PDXI-MF-16-400/14H|PDXI-MF-64-400/14L|PDXI-MF-64-400/14H|PDXI-MF-16-800/14L|PDXI-MF-16-800/14H|PDXI-MF-64-800/14L|PDXI-MF-64-800/14H|PDXI-MF-16-2M/14L|PDXI-MF-16-2M/14H|PDXI-MF-64-2M/14L|PDXI-MF-64-2M/14H),edit,edit,edit,edit,edit
      mask Display: disp('PDXI-MF-16-400/14L\nUEI\nDigital Output');port_label('input',1,'1');
  PDXI-MF 16bit series : S-Function  InitFcn=muei  FunctionName=doueipd2mfx  Parameters=channel, reset, initValue, sampletime, pcislot, boardType, board, devName  mask(ueipdximf16_do_6){boardtypein=PDXI-MF-16-333/16H, channel=[1], reset=[1], initValue=[0], sampletime=0.001, pcislot=-1}
      mask prompts: boardtypein "Board type:"; channel "Channel vector:"; reset "Reset vector:"; initValue "Initial value vector:"; pcislot "PCI slot (-1: autosearch):"
      mask help:
      | PDXI-MF 16bit series
      | United Electronic Industries
      | Digital Output
      mask init: same as xpcueilib/Digital Output/PD2-AO series
      mask Help: helpview(fullfile(docroot, 'mapfiles', 'xpc.map'), 'UEI_PDXI-MF-16bit-series_DOUT')
      mask StyleString: popup(PDXI-MF-16-50/16L|PDXI-MF-16-50/16H|PDXI-MF-64-50/16L|PDXI-MF-64-50/16H|PDXI-MF-16-150/16L|PDXI-MF-16-150/16H|PDXI-MF-64-150/16L|PDXI-MF-64-150/16H|PDXI-MF-16-333/16L|PDXI-MF-16-333/16H|PDXI-MF-64-333/16L|PDXI-MF-64-333/16H|PDXI-MF-16-500/16L|PDXI-MF-16-500/16H|PDXI-MF-64-500/16L|PDXI-MF-64-500/16H),edit,edit,edit,edit,edit
      mask Display: disp('PDXI-MF-16-333/16H\nUEI\nDigital Output');port_label('input',1,'1');
  PDXI-MFS 12bit series : S-Function  InitFcn=muei  FunctionName=doueipd2mfx  Parameters=channel, reset, initValue, sampletime, pcislot, boardType, board, devName  mask(ueipd2mfs12_do_6){boardtypein=PDXI-MFS-4-1M/12, channel=[1], reset=[1], initValue=[0], sampletime=0.001, pcislot=-1}
      mask prompts: boardtypein "Board type:"; channel "Channel vector:"; reset "Reset vector:"; initValue "Initial value vector:"; pcislot "PCI slot (-1: autosearch):"
      mask help:
      | PD2-MFS 12bit series
      | United Electronic Industries
      | Digital Output
      mask init: same as xpcueilib/Digital Output/PD2-AO series
      mask Help: helpview(fullfile(docroot, 'mapfiles', 'xpc.map'), 'UEI_PDXI-MFS-12bit-series_DOUT')
      mask StyleString: popup(PDXI-MFS-4-1M/12|PDXI-MFS-4-1M/12DG|PDXI-MFS-4-1M/12H|PDXI-MFS-8-1M/12|PDXI-MFS-8-1M/12DG|PDXI-MFS-8-1M/12H),edit,edit,edit,edit,edit
      mask Display: disp('PDXI-MFS-4-1M/12\nUEI\nDigital Output');port_label('input',1,'1');
  PDXI-MFS 14bit series : S-Function  InitFcn=muei  FunctionName=doueipd2mfx  Parameters=channel, reset, initValue, sampletime, pcislot, boardType, board, devName  mask(ueipd2mfs14_do_6){boardtypein=PDXI-MFS-4-500/14, channel=[1], reset=[1], initValue=[0], sampletime=0.001, pcislot=-1}
      mask prompts: boardtypein "Board type:"; channel "Channel vector:"; reset "Reset vector:"; initValue "Initial value vector:"; pcislot "PCI slot (-1: autosearch):"
      mask help:
      | PD2-MFS 14bit series
      | United Electronic Industries
      | Digital Output
      mask init: same as xpcueilib/Digital Output/PD2-AO series
      mask Help: helpview(fullfile(docroot, 'mapfiles', 'xpc.map'), 'UEI_PDXI-MFS-14bit-series_DOUT')
      mask StyleString: popup(PDXI-MFS-4-500/14|PDXI-MFS-4-500/14DG|PDXI-MFS-4-500/14H|PDXI-MFS-8-500/14|PDXI-MFS-8-500/14DG|PDXI-MFS-8-500/14H|PDXI-MFS-4-800/14|PDXI-MFS-4-800/14DG|PDXI-MFS-4-800/14H|PDXI-MFS-8-800/14|PDXI-MFS-8-800/14DG|PDXI-MFS-8-800/14H|PDXI-MFS-4-2M/14|PDXI-MFS-4-2M/14DG|PDXI-MFS-4-2M/14H|PDXI-MFS-8-2M/14|PDXI-MFS-8-2M/14DG|PDXI-MFS-8-2M/14H),edit,edit,edit,edit,edit
      mask Display: disp('PDXI-MFS-4-500/14\nUEI\nDigital Output');port_label('input',1,'1');
  PDXI-MFS 16bit series : S-Function  InitFcn=muei  FunctionName=doueipd2mfx  Parameters=channel, reset, initValue, sampletime, pcislot, boardType, board, devName  mask(ueipd2mfs16_do_6){boardtypein=PDXI-MFS-4-300/16, channel=[1], reset=[1], initValue=[0], sampletime=0.001, pcislot=-1}
      mask prompts: boardtypein "Board type:"; channel "Channel vector:"; reset "Reset vector:"; initValue "Initial value vector:"; pcislot "PCI slot (-1: autosearch):"
      mask help:
      | PD2-MFS 16bit series
      | United Electronic Industries
      | Digital Output
      mask init: same as xpcueilib/Digital Output/PD2-AO series
      mask Help: helpview(fullfile(docroot, 'mapfiles', 'xpc.map'), 'UEI_PDXI-MFS-16bit-series_DOUT')
      mask StyleString: popup(PDXI-MFS-4-300/16|PDXI-MFS-4-300/16DG|PDXI-MFS-4-300/16H|PDXI-MFS-8-300/16|PDXI-MFS-8-300/16DG|PDXI-MFS-8-300/16H|PDXI-MFS-4-500/16|PDXI-MFS-4-500/16DG|PDXI-MFS-4-500/16H|PDXI-MFS-8-500/16|PDXI-MFS-8-500/16DG|PDXI-MFS-8-500/16H),edit,edit,edit,edit,edit
      mask Display: disp('PDXI-MFS-4-300/16\nUEI\nDigital Output');port_label('input',1,'1');
